simulink model "simulation_DICBF"  (R2022a)
settings: Solver=VariableStepAuto  StartTime=0.0  StopTime=simTime  FixedStep=0.01  RelTol=1e-3
values from neighbouring files (symbols this model uses):
  Kd = 1    [setup.m]    (also in setup_DICBF.m)
  Kp = 0.2    [setup.m]    (also in setup_DICBF.m)
  M = 1*eye(2)    [setup.m]    (also in setup_DICBF.m)
  mu = 1    [setup.m]    (also in setup_DICBF.m = 0.8)
  obs = [qO1 qO2]    [setup.m]
  qdotstart = [0,0]    [setup.m]    (also in setup_DICBF.m = [0 ; 0])
  qg = [4, -1]    [setup.m]    (also in setup_DICBF.m)
  qstart = [0,0]    [setup.m]    (also in setup_DICBF.m = [0 ; 0])
  r = [r1 r1 0.5 0.05 0.05]    [setup.m]
  threshold_skip = 0.0    (= 0)    [setup.m]    (also in setup_DICBF.m = 0.1)
undefined symbols (not defined in the file or in its folder): conditional_delta
libraries: slctrlblks x1
settings Model: Creator=mirkomizzoni  LastModifiedBy=mirkomizzoni

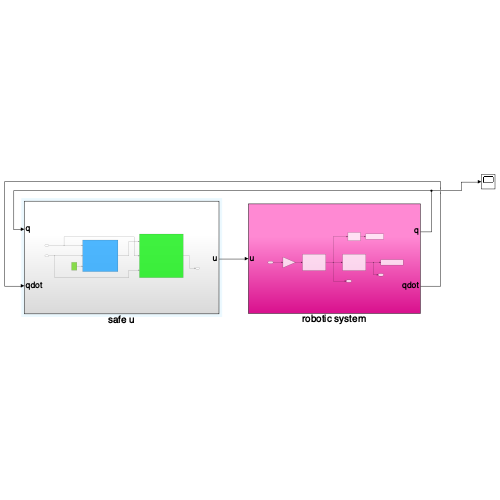
[thumbnail: Simulink's stored preview of the top-level diagram]
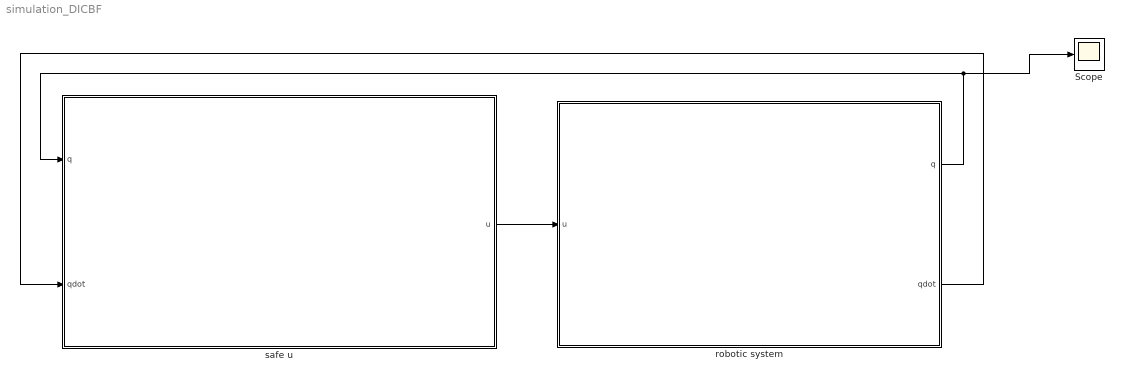
== system simulation_DICBF ==
  Scope : Scope
  robotic system : Subsystem
  safe u : Subsystem
  wires:
  safe u/1(u) -> robotic system/1(u)
  robotic system/1(q) -> Scope/1, safe u/1(q)
  robotic system/2(qdot) -> safe u/2(qdot)

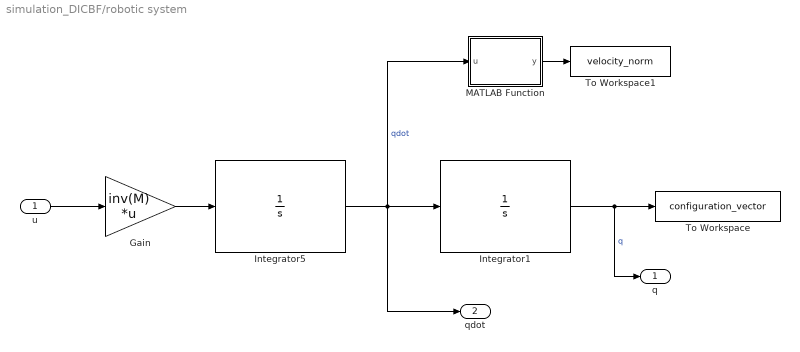
== system simulation_DICBF/robotic system ==
  u : Inport
  Gain : Gain  Gain=inv(M)  Multiplication=Matrix(K*u)
  Integrator1 : Integrator  InitialCondition=qstart
  Integrator5 : Integrator  InitialCondition=qdotstart
  MATLAB Function : MATLAB Function  TreatAsAtomicUnit=on
  To Workspace : ToWorkspace  VariableName=configuration_vector  SaveFormat=Timeseries  SampleTime=0.01
  To Workspace1 : ToWorkspace  VariableName=velocity_norm  SaveFormat=Timeseries  SampleTime=0.01
  q : Outport
  qdot : Outport  Port=2
  wires:
  Integrator5/1 -> qdot/1, MATLAB Function/1(u), Integrator1/1  "qdot"
  Integrator1/1 -> q/1, To Workspace/1  "q"
  MATLAB Function/1(y) -> To Workspace1/1
  Gain/1 -> Integrator5/1
  u/1 -> Gain/1

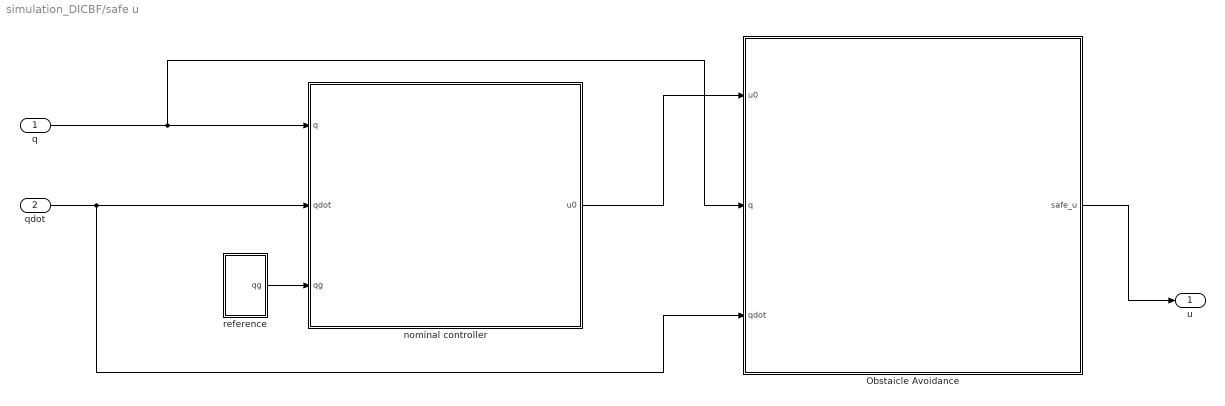
== system simulation_DICBF/safe u ==
  q : Inport
  qdot : Inport  Port=2
  Obstaicle Avoidance : Subsystem
  nominal controller : Subsystem
  reference : Subsystem
  u : Outport
  wires:
  reference/1(qg) -> nominal controller/3(qg)
  nominal controller/1(u0) -> Obstaicle Avoidance/1(u0)
  Obstaicle Avoidance/1(safe_u) -> u/1
  q/1 -> Obstaicle Avoidance/2(q), nominal controller/1(q)
  qdot/1 -> Obstaicle Avoidance/3(qdot), nominal controller/2(qdot)

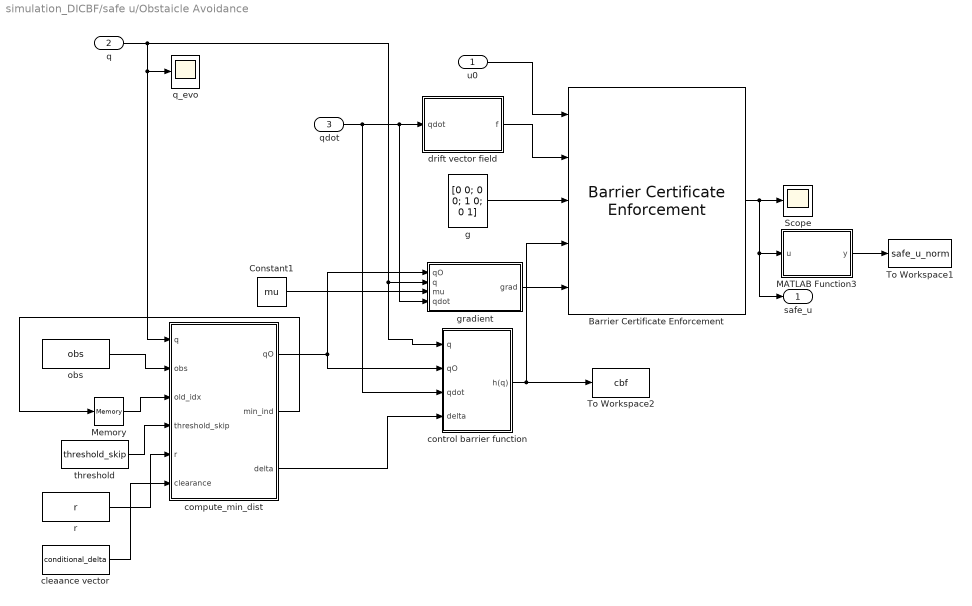
== system simulation_DICBF/safe u/Obstaicle Avoidance ==
  u0 : Inport
  q : Inport  Port=2
  qdot : Inport  Port=3
  Barrier Certificate Enforcement : slctrlblks/Barrier Certificate Enforcement  nx=4  nu=2  nc=1  gamma=alpha  beta=1  external_umax=off  external_umin=off  Ts=0.01  maxiter=200  tol=1e-06  output_exitflag=off
      settings: SourceProductBaseCode=SD
  Constant1 : Constant  Value=mu
  MATLAB Function3 : MATLAB Function  TreatAsAtomicUnit=on
  Memory : Memory  InitialCondition=1
  Scope : Scope
  To Workspace1 : ToWorkspace  VariableName=safe_u_norm  SaveFormat=Timeseries  SampleTime=0.01
  To Workspace2 : ToWorkspace  VariableName=cbf  SaveFormat=Timeseries  SampleTime=0.01
  cleaance vector : Constant  Value=conditional_delta
  compute_min_dist : MATLAB Function  TreatAsAtomicUnit=on
  control barrier function : Subsystem
  drift vector field : MATLAB Function  TreatAsAtomicUnit=on
  g : Constant  Value=[0 0; 0 0; 1 0; 0 1]  VectorParams1D=off
  gradient : MATLAB Function  TreatAsAtomicUnit=on
  obs : Constant  Value=obs  VectorParams1D=off
  q_evo : Scope
  r : Constant  Value=r
  threshold : Constant  Value=threshold_skip  VectorParams1D=off
  safe_u : Outport
  wires:
  q/1 -> q_evo/1, compute_min_dist/1(q), control barrier function/1(q), gradient/2(q)
  compute_min_dist/1(qO) -> control barrier function/2(qO), gradient/1(qO)
  qdot/1 -> gradient/4(qdot), drift vector field/1(qdot), control barrier function/3(qdot)
  control barrier function/1(h(q)) -> Barrier Certificate Enforcement/4, To Workspace2/1
  MATLAB Function3/1(y) -> To Workspace1/1
  threshold/1 -> compute_min_dist/4(threshold_skip)
  u0/1 -> Barrier Certificate Enforcement/1
  obs/1 -> compute_min_dist/2(obs)
  g/1 -> Barrier Certificate Enforcement/3
  gradient/1(grad) -> Barrier Certificate Enforcement/5
  Constant1/1 -> gradient/3(mu)
  Memory/1 -> compute_min_dist/3(old_idx)
  drift vector field/1(f) -> Barrier Certificate Enforcement/2
  r/1 -> compute_min_dist/5(r)
  Barrier Certificate Enforcement/1 -> MATLAB Function3/1(u), safe_u/1, Scope/1
  compute_min_dist/2(min_ind) -> Memory/1
  compute_min_dist/3(delta) -> control barrier function/4(delta)
  cleaance vector/1 -> compute_min_dist/6(clearance)

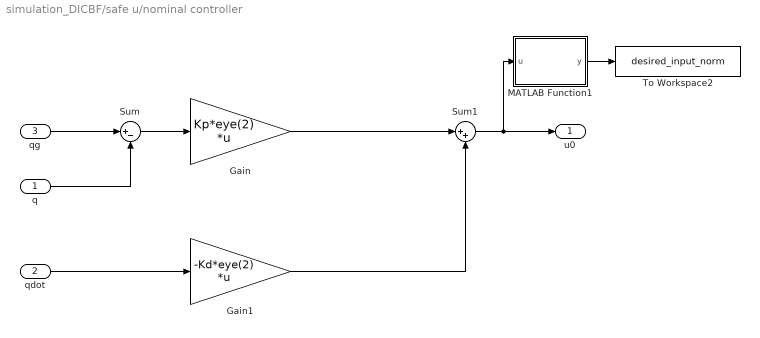
== system simulation_DICBF/safe u/nominal controller ==
  q : Inport
  qdot : Inport  Port=2
  qg : Inport  Port=3
  Gain : Gain  Gain=Kp*eye(2)  Multiplication=Matrix(K*u)
  Gain1 : Gain  Gain=-Kd*eye(2)  Multiplication=Matrix(K*u)
  MATLAB Function1 : MATLAB Function  TreatAsAtomicUnit=on
  Sum : Sum  Inputs=|+-
  Sum1 : Sum  Inputs=|++
  To Workspace2 : ToWorkspace  VariableName=desired_input_norm  SaveFormat=Timeseries  SampleTime=0.01
  u0 : Outport
  wires:
  MATLAB Function1/1(y) -> To Workspace2/1
  q/1 -> Sum/2
  qg/1 -> Sum/1
  Sum/1 -> Gain/1
  Gain/1 -> Sum1/1
  qdot/1 -> Gain1/1
  Gain1/1 -> Sum1/2
  Sum1/1 -> MATLAB Function1/1(u), u0/1

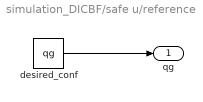
== system simulation_DICBF/safe u/reference ==
  desired_conf : Constant  Value=qg
  qg : Outport
  wires:
  desired_conf/1 -> qg/1

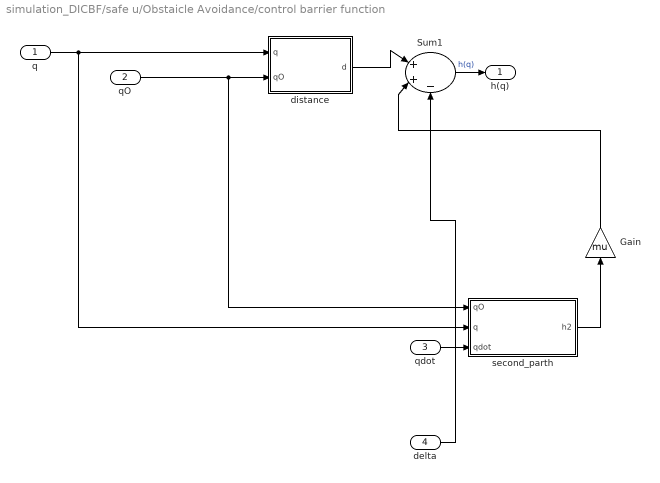
== system simulation_DICBF/safe u/Obstaicle Avoidance/control barrier function ==
  q : Inport
  qO : Inport  Port=2
  qdot : Inport  Port=3
  delta : Inport  Port=4
  Gain : Gain  Gain=mu
  Sum1 : Sum  Inputs=|++-
  distance : MATLAB Function  TreatAsAtomicUnit=on
  second_parth : MATLAB Function  TreatAsAtomicUnit=on
  h(q) : Outport
  wires:
  delta/1 -> Sum1/3
  q/1 -> distance/1(q), second_parth/2(q)
  qdot/1 -> second_parth/3(qdot)
  second_parth/1(h2) -> Gain/1
  qO/1 -> second_parth/1(qO), distance/2(qO)
  Sum1/1 -> h(q)/1  "h(q)"
  distance/1(d) -> Sum1/1
  Gain/1 -> Sum1/2

== matlab function simulation_DICBF/safe u/Obstaicle Avoidance/gradient ==
  data: qO input; grad output; q input; mu input; qdot input
function grad = gradient(qO,q, mu, qdot)
   gradp = 2*(q-qO)'+mu*qdot';
   grapdot = mu * (q-qO)';
   grad = [gradp, grapdot]; 
end

== matlab function simulation_DICBF/safe u/Obstaicle Avoidance/control barrier function/distance ==
  data: q input; qO input; d output
function d = distance(q,qO)
    d = norm(q-qO);
end

== matlab function simulation_DICBF/safe u/Obstaicle Avoidance/compute_min_dist ==
  data: q input; obs input; qO output; min_ind output; old_idx input; threshold_skip input; r input; delta output; clearance input
function [qO,min_ind,delta] = min_dist(q, obs, old_idx, threshold_skip, r, clearance)
[~,n] = size(obs);
min = norm(q-obs(:,1))-r(1)-clearance(1);
min_ind = 1;
for i=2:n
    t = norm(q-obs(:,i))-r(i)-clearance(i);
    if t<min
        min_ind = i;
        min = t;
    end
end

old_dist = norm(q-obs(:,old_idx))-r(old_idx)-clearance(old_idx);
if abs(old_dist-min) < threshold_skip
    qO = obs(:,old_idx);
    min_ind = old_idx;
else
    qO = obs(:,min_ind);
end
rn = r(min_ind);
cn = clearance(min_ind);
delta = rn+cn;
end

== matlab function simulation_DICBF/robotic system/MATLAB Function ==
  data: u input; y output
function y = norm_func(u)
        
y = norm(u);

== matlab function simulation_DICBF/safe u/Obstaicle Avoidance/MATLAB Function3 ==
  data: u input; y output
function y = norm_func(u)
        
y = norm(u);

== matlab function simulation_DICBF/safe u/Obstaicle Avoidance/control barrier function/second_parth ==
  data: qO input; h2 output; q input; qdot input
function h2 = second_parth(qO,q,qdot)
   h2 = (q-qO)'*qdot;
end

== matlab function simulation_DICBF/safe u/Obstaicle Avoidance/drift vector field ==
  data: qdot input; f output
function f = make_f(qdot)
    f = [qdot; 0; 0];
end

== matlab function simulation_DICBF/safe u/nominal controller/MATLAB Function1 ==
  data: u input; y output
function y = norm_func(u)
        
y = norm(u);
